simulink model "week1_problem5_2005052"  (R2020b)
settings: Solver=VariableStepAuto  StartTime=0.0  StopTime=10.0  RelTol=1e-3
settings Model: Creator=admin  LastModifiedBy=admin

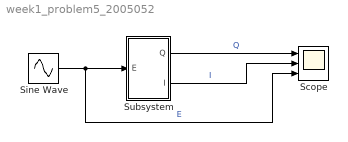
== system week1_problem5_2005052 ==
  Scope : Scope  NumInputPorts=3
  Sine Wave : Sin  Frequency=5  SampleTime=0
  Subsystem : Subsystem  mask{C=10^-5, R=10}
  wires:
  Subsystem/2(I) -> Scope/2  "I"
  Subsystem/1(Q) -> Scope/1  "Q"
  Sine Wave/1 -> Scope/3, Subsystem/1(E)  "E"

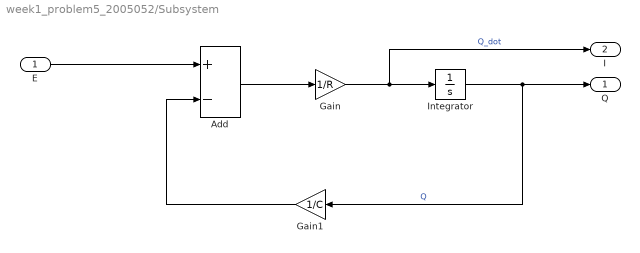
== system week1_problem5_2005052/Subsystem ==
  E : Inport
  Add : Sum  Inputs=+-
  Gain : Gain  Gain=1/R
  Gain1 : Gain  Gain=1/C
  Integrator : Integrator
  Q : Outport
  I : Outport  Port=2
  wires:
  Integrator/1 -> Q/1, Gain1/1  "Q"
  Add/1 -> Gain/1
  Gain1/1 -> Add/2
  Gain/1 -> I/1, Integrator/1  "Q_dot"
  E/1 -> Add/1
